simulink library "HeatTransfer2Ground_Simple"  (R2018b)
settings: Solver=ode45  StartTime=0.0  StopTime=10.0  RelTol=1e-3  EnableMultiTasking=on
settings Model: Creator=drhf  LastModifiedBy=drhf
settings DataIOCC: LimitDataPoints=on  SaveFormat=Array  SignalLoggingSaveFormat=ModelDataLogs
settings OptimizationCC: ExpressionDepthLimit=2147483647  LifeSpan=inf
settings DebuggingCC: UnderspecifiedInitializationDetection=Classic  MergeDetectMultiDrivingBlocksExec=none  SolverPrmCheckMsg=warning  FcnCallInpInsideContextMsg=warning  StateNameClashWarn=warning  SFUnexpectedBacktrackingDiag=warning  SFNoUnconditionalDefaultTransitionDiag=warning  SFExecutionAtInitializationDiag=none
settings HardwareCC: ProdBitPerPointer=32  ProdBitPerSizeT=32  ProdBitPerPtrDiffT=32  ProdLargestAtomicFloat=None  ProdIntDivRoundTo=Undefined  ProdEndianess=Unspecified  ProdWordSize=32  ProdHWDeviceType=32-bit Generic
settings ModelReferenceCC: PropagateSignalLabelsOutOfModel=off
settings SFSimCC: SimUseLocalCustomCode=off
settings RTWCC: RTWUseLocalCustomCode=off
settings CodeAppCC: StateflowObjectComments=on
settings GRTTargetCC: TargetLangStandard=C89/C90 (ANSI)  GeneratePreprocessorConditionals=Disable all  CombineOutputUpdateFcns=off  GRTInterface=on
settings ConfigComp: CovMetricSettings=dw  CovHtmlReporting=on  CovSaveCumulativeToWorkspaceVar=on  CovSaveSingleToWorkspaceVar=on  CovExternalEMLEnable=off

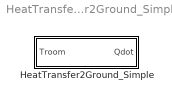
== system HeatTransfer2Ground_Simple ==
  HeatTransfer2Ground_Simple : Subsystem  mask(Heat Transfer to Ground simple Model){Tground=10, UAground=0.2*70}
      mask prompts: Tground "Ground temperature in °C"; UAground "Heat transfer to ground in W/K"
      mask help:
      | Very simple model for the heat transfer of a house to the ground.
      | See Help for details.
      mask Help: web(fullfile(path_carnot('help'),'Heattransfer2Ground_Simple.html'),'-helpbrowser')

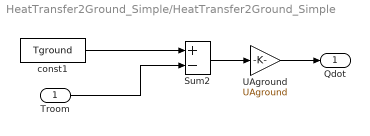
== system HeatTransfer2Ground_Simple/HeatTransfer2Ground_Simple ==
  Troom : Inport
  Sum2 : Sum  Inputs=+-  SaturateOnIntegerOverflow=on  InputSameDT=on  OutDataTypeStr=Inherit: Same as first input
  UAground : Gain  Gain=UAground  SaturateOnIntegerOverflow=on  OutDataTypeStr=Inherit: Same as input  ParamDataTypeStr=Inherit: Same as input
  const1 : Constant  Value=Tground
  Qdot : Outport
  wires:
  Troom/1 -> Sum2/2
  UAground/1 -> Qdot/1
  const1/1 -> Sum2/1
  Sum2/1 -> UAground/1
